simulink model "ifk_updated_armpi_fpv"  (R2023b)
settings: Solver=VariableStepAuto  StartTime=0.0001  StopTime=10.0  RelTol=1e-3
libraries: slpidlib x6
settings Model: Creator=15404  LastModifiedBy=PC
settings SolverCC: AlgebraicLoopSolver=TrustRegion
settings DebuggingCC: UnconnectedInputMsg=warning  UnconnectedOutputMsg=warning  UnconnectedLineMsg=warning
settings ModelReferenceCC: EnableRefExpFcnMdlSchedulingChecks=on
settings RTWCC: DLArmComputeVersion=19.05

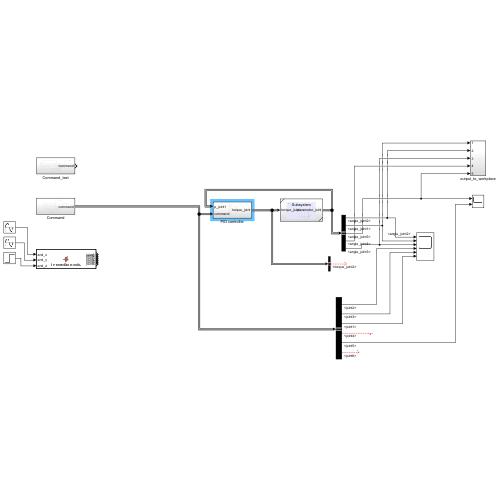
[thumbnail: Simulink's stored preview of the top-level diagram]
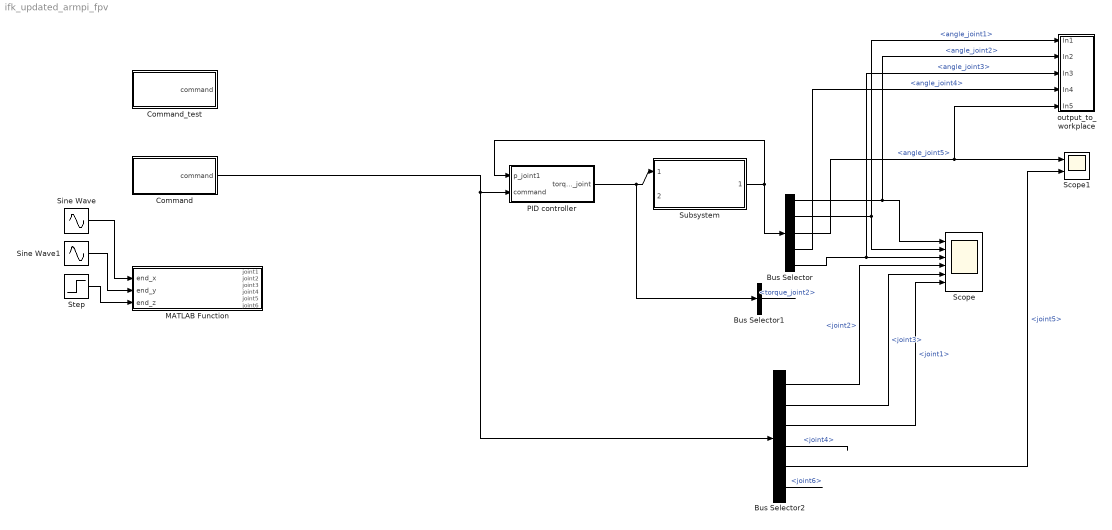
== system ifk_updated_armpi_fpv ==
  Bus Selector : BusSelector  OutputSignals=angle_joint2,angle_joint1,angle_joint5,angle_joint4,angle_joint3
  Bus Selector1 : BusSelector  OutputSignals=torque_joint2
  Bus Selector2 : BusSelector  OutputSignals=joint2,joint3,joint1,joint4,joint5,joint6
  Command : Subsystem
  Command_test : Subsystem
  MATLAB Function : MATLAB Function  TreatAsAtomicUnit=on
  PID controller : Subsystem
  Scope : Scope  NumInputPorts=6
  Scope1 : Scope  NumInputPorts=2
  Sine Wave : Sin  Amplitude=0.2  Phase=pi/2  SampleTime=0
  Sine Wave1 : Sin  Amplitude=0.2  SampleTime=0
  Step : Step  Time=0  After=0.1  SampleTime=0
  Subsystem : Subsystem  ReferencedSubsystem=Subsystem
  output_to_workplace : Subsystem
  wires:
  PID controller/1(torque_joint) -> Bus Selector1/1, Subsystem/1
  Subsystem/1 -> Bus Selector/1, PID controller/1(p_joint1)
  Bus Selector/1 -> output_to_workplace/2(In2), Scope/1  "<angle_joint2>"
  Bus Selector1/1 -> ?  "<torque_joint2>"
  Bus Selector/2 -> Scope/2, output_to_workplace/1(In1)  "<angle_joint1>"
  Bus Selector/3 -> output_to_workplace/5(In5), Scope1/1  "<angle_joint5>"
  Bus Selector/5 -> output_to_workplace/3(In3), Scope/3  "<angle_joint3>"
  Command/1(command) -> Bus Selector2/1, PID controller/2(command)
  Bus Selector2/1 -> Scope/4  "<joint2>"
  Bus Selector2/2 -> Scope/5  "<joint3>"
  Bus Selector2/3 -> Scope/6  "<joint1>"
  Bus Selector/4 -> output_to_workplace/4(In4)  "<angle_joint4>"
  Bus Selector2/4 -> ?  "<joint4>"
  Bus Selector2/5 -> Scope1/2  "<joint5>"
  Step/1 -> MATLAB Function/3(end_z)
  Sine Wave1/1 -> MATLAB Function/2(end_y)
  Sine Wave/1 -> MATLAB Function/1(end_x)
  Bus Selector2/6 -> ?  "<joint6>"

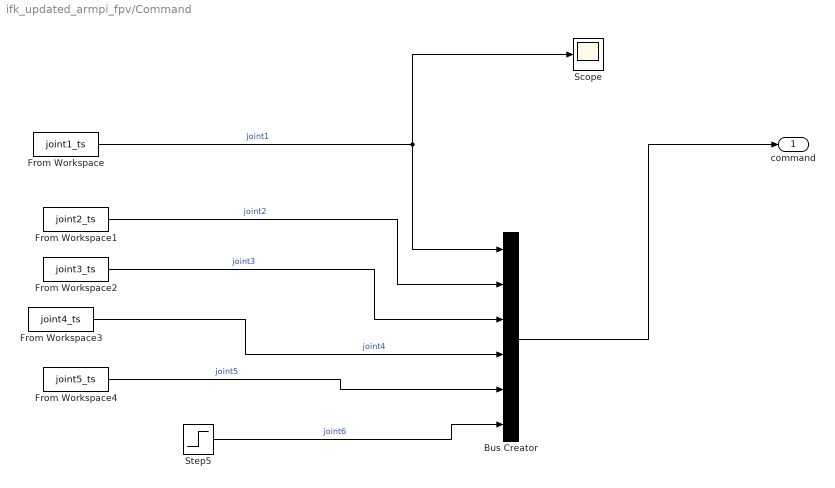
== system ifk_updated_armpi_fpv/Command ==
  Bus Creator : BusCreator  Inputs=6
  From Workspace : FromWorkspace  VariableName=joint1_ts
  From Workspace1 : FromWorkspace  VariableName=joint2_ts
  From Workspace2 : FromWorkspace  VariableName=joint3_ts
  From Workspace3 : FromWorkspace  VariableName=joint4_ts
  From Workspace4 : FromWorkspace  VariableName=joint5_ts
  Scope : Scope
  Step5 : Step  After=0  SampleTime=0
  command : Outport
  wires:
  Bus Creator/1 -> command/1
  From Workspace/1 -> Scope/1, Bus Creator/1  "joint1"
  From Workspace2/1 -> Bus Creator/3  "joint3"
  From Workspace3/1 -> Bus Creator/4  "joint4"
  From Workspace4/1 -> Bus Creator/5  "joint5"
  Step5/1 -> Bus Creator/6  "joint6"
  From Workspace1/1 -> Bus Creator/2  "joint2"

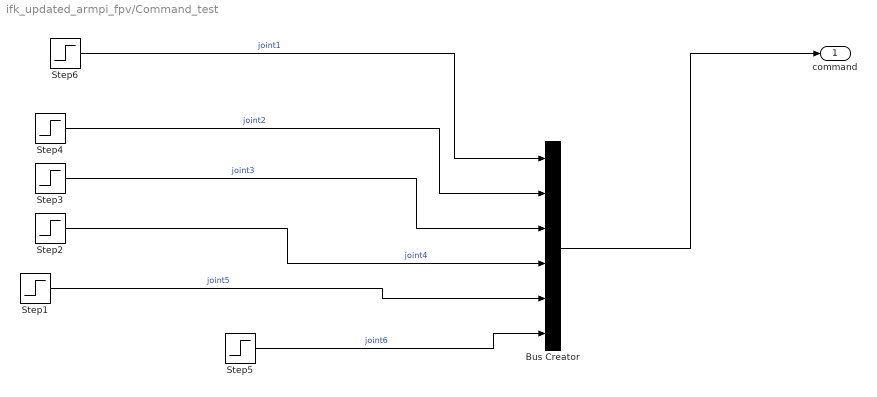
== system ifk_updated_armpi_fpv/Command_test ==
  Bus Creator : BusCreator  Inputs=6
  Step{1..6} (6 alike) : Step  After=0*pi/180  SampleTime=0
  command : Outport
  wires:
  Bus Creator/1 -> command/1
  Step6/1 -> Bus Creator/1  "joint1"
  Step3/1 -> Bus Creator/3  "joint3"
  Step2/1 -> Bus Creator/4  "joint4"
  Step1/1 -> Bus Creator/5  "joint5"
  Step5/1 -> Bus Creator/6  "joint6"
  Step4/1 -> Bus Creator/2  "joint2"

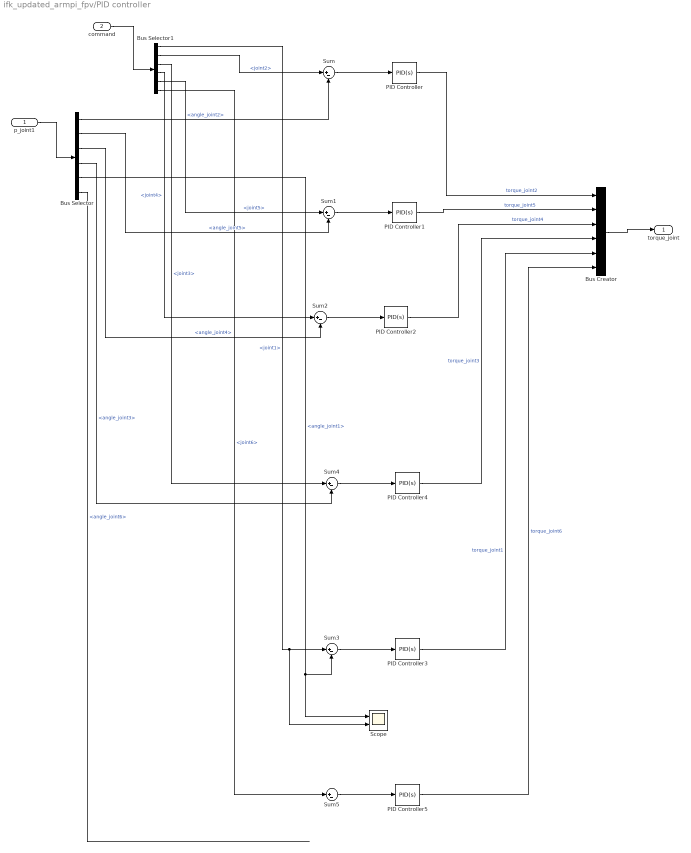
== system ifk_updated_armpi_fpv/PID controller ==
  p_joint1 : Inport
  command : Inport  Port=2
  Bus Creator : BusCreator  Inputs=6
  Bus Selector : BusSelector  OutputSignals=angle_joint2,angle_joint5,angle_joint4,angle_joint3,angle_joint1,angle_joint6
  Bus Selector1 : BusSelector  OutputSignals=joint1,joint2,joint3,joint4,joint5,joint6
  PID Controller : slpidlib/PID Controller  Controller=PID  Form=Parallel  TimeDomain=Continuous-time  UseExternalTs=off  SampleTime=-1  IntegratorMethod=Forward Euler  FilterMethod=Forward Euler  ControllerParametersSource=internal  P=5  I=500  UseKiTs=off  D=0.1  N=100  UseFilter=on  TunerSelectOption=Transfer Function Based (PID Tuner App)  InitialConditionSource=internal  InitialConditionForIntegrator=0  InitialConditionForFilter=0  DifferentiatorICPrevScaledInput=0  ExternalReset=none  TrackingMode=off  Kt=1  LimitOutput=off  SatLimitsSource=internal  UpperSaturationLimit=inf  LowerSaturationLimit=-inf  LinearizeAsGain=on  AntiWindupMode=none  Kb=1  LimitIntegrator=off  UpperIntegratorSaturationLimit=inf  LowerIntegratorSaturationLimit=-inf  POutMin=[]  POutMax=[]  IOutMin=[]  IOutMax=[]  DOutMin=[]  DOutMax=[]  NOutMin=[]  NOutMax=[]  SumOutMin=[]  SumOutMax=[]  SaturationOutMin=[]  SaturationOutMax=[]  PParamMin=[]  PParamMax=[]  IParamMin=[]  IParamMax=[]  DParamMin=[]  DParamMax=[]  NParamMin=[]  NParamMax=[]  KbParamMin=[]  KbParamMax=[]  KtParamMin=[]  KtParamMax=[]  KbOutMin=[]  KbOutMax=[]  KtOutMin=[]  KtOutMax=[]  IntegratorOutMin=[]  IntegratorOutMax=[]  FilterOutMin=[]  FilterOutMax=[]  SumI1OutMin=[]  SumI1OutMax=[]  SumI2OutMin=[]  SumI2OutMax=[]  SumI3OutMin=[]  SumI3OutMax=[]  SumI4OutMin=[]  SumI4OutMax=[]  SumDOutMin=[]  SumDOutMax=[]  DifferentiatorOutMin=[]  DifferentiatorOutMax=[]  FilterDiffOutCoefMin=[]  FilterDiffOutCoefMax=[]  ReciprocalOutMin=[]  ReciprocalOutMax=[]  SumDenOutMin=[]  SumDenOutMax=[]  SumNumOutMin=[]  SumNumOutMax=[]  DivideOutMin=[]  DivideOutMax=[]  UdiffTsProdOutMin=[]  UdiffTsProdOutMax=[]  NTsProdOutMin=[]  NTsProdOutMax=[]  UintegralTsProdOutMin=[]  UintegralTsProdOutMax=[]  UngainTsProdOutMin=[]  UngainTsProdOutMax=[]  ClampingZeroOutDataTypeStr=Inherit: Inherit via back propagation  ClampingZeroOutMin=[]  ClampingZeroOutMax=[]  FilterDenConstantOutDataTypeStr=Inherit: Inherit via back propagation  FilterDenConstantOutMin=[]  FilterDenConstantOutMax=[]  PCopyOutDataTypeStr=Inherit: Inherit via back propagation  PCopyOutMin=[]  PCopyOutMax=[]  NCopyOutDataTypeStr=Inherit: Inherit via back propagation  NCopyOutMin=[]  NCopyOutMax=[]  IntegratorContinuousStateAttributes=''  IntegratorStateMustResolveToSignalObject=off  IntegratorRTWStateStorageClass=Auto  FilterContinuousStateAttributes=''  FilterStateMustResolveToSignalObject=off  FilterRTWStateStorageClass=Auto  ParallelPVariant=InternalParameters  IdealPVariant=Disabled  IVariant=InternalParameters  DVariant=InternalParameters  IntegratorVariant=Continuous  SatVariant=Disabled  AWVariant=Passthrough  PCopyVariant=Disabled  TRVariant=Disabled  FdbkBlocksVariant=Forward  IdealPFdbkVariant=Disabled  SatFdbkVariant=Disabled  DerivativeFilterVariant=ContFilter  NVariant=InternalParameters  NCopyVariant=Disabled  FilterICVariant=InternalICsFilter  IntegratorICVariant=InternalICs  ExternalResetVariant=Disabled  TRSumVariant=Passthrough  SumFdbkVariant=Disabled  SumVariant=Sum_PID  TsampFilterVariant=InternalTs  TsampNgainVariant=Passthrough  TsampIntegralVariant=Disabled_SignalSpec  ExternalSaturationOutDataTypeStr=Inherit: Same as second input
  PID Controller{1..4} (4 alike) : slpidlib/PID Controller  Controller=PID  Form=Parallel  TimeDomain=Continuous-time  UseExternalTs=off  SampleTime=-1  IntegratorMethod=Forward Euler  FilterMethod=Forward Euler  ControllerParametersSource=internal  P=1  I=50  UseKiTs=off  D=0.1  N=100  UseFilter=on  TunerSelectOption=Transfer Function Based (PID Tuner App)  InitialConditionSource=internal  InitialConditionForIntegrator=0  InitialConditionForFilter=0  DifferentiatorICPrevScaledInput=0  ExternalReset=none  TrackingMode=off  Kt=1  LimitOutput=off  SatLimitsSource=internal  UpperSaturationLimit=inf  LowerSaturationLimit=-inf  LinearizeAsGain=on  AntiWindupMode=none  Kb=1  LimitIntegrator=off  UpperIntegratorSaturationLimit=inf  LowerIntegratorSaturationLimit=-inf  POutMin=[]  POutMax=[]  IOutMin=[]  IOutMax=[]  DOutMin=[]  DOutMax=[]  NOutMin=[]  NOutMax=[]  SumOutMin=[]  SumOutMax=[]  SaturationOutMin=[]  SaturationOutMax=[]  PParamMin=[]  PParamMax=[]  IParamMin=[]  IParamMax=[]  DParamMin=[]  DParamMax=[]  NParamMin=[]  NParamMax=[]  KbParamMin=[]  KbParamMax=[]  KtParamMin=[]  KtParamMax=[]  KbOutMin=[]  KbOutMax=[]  KtOutMin=[]  KtOutMax=[]  IntegratorOutMin=[]  IntegratorOutMax=[]  FilterOutMin=[]  FilterOutMax=[]  SumI1OutMin=[]  SumI1OutMax=[]  SumI2OutMin=[]  SumI2OutMax=[]  SumI3OutMin=[]  SumI3OutMax=[]  SumI4OutMin=[]  SumI4OutMax=[]  SumDOutMin=[]  SumDOutMax=[]  DifferentiatorOutMin=[]  DifferentiatorOutMax=[]  FilterDiffOutCoefMin=[]  FilterDiffOutCoefMax=[]  ReciprocalOutMin=[]  ReciprocalOutMax=[]  SumDenOutMin=[]  SumDenOutMax=[]  SumNumOutMin=[]  SumNumOutMax=[]  DivideOutMin=[]  DivideOutMax=[]  UdiffTsProdOutMin=[]  UdiffTsProdOutMax=[]  NTsProdOutMin=[]  NTsProdOutMax=[]  UintegralTsProdOutMin=[]  UintegralTsProdOutMax=[]  UngainTsProdOutMin=[]  UngainTsProdOutMax=[]  ClampingZeroOutDataTypeStr=Inherit: Inherit via back propagation  ClampingZeroOutMin=[]  ClampingZeroOutMax=[]  FilterDenConstantOutDataTypeStr=Inherit: Inherit via back propagation  FilterDenConstantOutMin=[]  FilterDenConstantOutMax=[]  PCopyOutDataTypeStr=Inherit: Inherit via back propagation  PCopyOutMin=[]  PCopyOutMax=[]  NCopyOutDataTypeStr=Inherit: Inherit via back propagation  NCopyOutMin=[]  NCopyOutMax=[]  IntegratorContinuousStateAttributes=''  IntegratorStateMustResolveToSignalObject=off  IntegratorRTWStateStorageClass=Auto  FilterContinuousStateAttributes=''  FilterStateMustResolveToSignalObject=off  FilterRTWStateStorageClass=Auto  ParallelPVariant=InternalParameters  IdealPVariant=Disabled  IVariant=InternalParameters  DVariant=InternalParameters  IntegratorVariant=Continuous  SatVariant=Disabled  AWVariant=Passthrough  PCopyVariant=Disabled  TRVariant=Disabled  FdbkBlocksVariant=Forward  IdealPFdbkVariant=Disabled  SatFdbkVariant=Disabled  DerivativeFilterVariant=ContFilter  NVariant=InternalParameters  NCopyVariant=Disabled  FilterICVariant=InternalICsFilter  IntegratorICVariant=InternalICs  ExternalResetVariant=Disabled  TRSumVariant=Passthrough  SumFdbkVariant=Disabled  SumVariant=Sum_PID  TsampFilterVariant=InternalTs  TsampNgainVariant=Passthrough  TsampIntegralVariant=Disabled_SignalSpec  ExternalSaturationOutDataTypeStr=Inherit: Same as second input
  PID Controller5 : slpidlib/PID Controller  Controller=PID  Form=Parallel  TimeDomain=Continuous-time  UseExternalTs=off  SampleTime=-1  IntegratorMethod=Forward Euler  FilterMethod=Forward Euler  ControllerParametersSource=internal  P=1  I=5  UseKiTs=off  D=1  N=100  UseFilter=on  TunerSelectOption=Transfer Function Based (PID Tuner App)  InitialConditionSource=internal  InitialConditionForIntegrator=0  InitialConditionForFilter=0  DifferentiatorICPrevScaledInput=0  ExternalReset=none  TrackingMode=off  Kt=1  LimitOutput=off  SatLimitsSource=internal  UpperSaturationLimit=inf  LowerSaturationLimit=-inf  LinearizeAsGain=on  AntiWindupMode=none  Kb=1  LimitIntegrator=off  UpperIntegratorSaturationLimit=inf  LowerIntegratorSaturationLimit=-inf  POutMin=[]  POutMax=[]  IOutMin=[]  IOutMax=[]  DOutMin=[]  DOutMax=[]  NOutMin=[]  NOutMax=[]  SumOutMin=[]  SumOutMax=[]  SaturationOutMin=[]  SaturationOutMax=[]  PParamMin=[]  PParamMax=[]  IParamMin=[]  IParamMax=[]  DParamMin=[]  DParamMax=[]  NParamMin=[]  NParamMax=[]  KbParamMin=[]  KbParamMax=[]  KtParamMin=[]  KtParamMax=[]  KbOutMin=[]  KbOutMax=[]  KtOutMin=[]  KtOutMax=[]  IntegratorOutMin=[]  IntegratorOutMax=[]  FilterOutMin=[]  FilterOutMax=[]  SumI1OutMin=[]  SumI1OutMax=[]  SumI2OutMin=[]  SumI2OutMax=[]  SumI3OutMin=[]  SumI3OutMax=[]  SumI4OutMin=[]  SumI4OutMax=[]  SumDOutMin=[]  SumDOutMax=[]  DifferentiatorOutMin=[]  DifferentiatorOutMax=[]  FilterDiffOutCoefMin=[]  FilterDiffOutCoefMax=[]  ReciprocalOutMin=[]  ReciprocalOutMax=[]  SumDenOutMin=[]  SumDenOutMax=[]  SumNumOutMin=[]  SumNumOutMax=[]  DivideOutMin=[]  DivideOutMax=[]  UdiffTsProdOutMin=[]  UdiffTsProdOutMax=[]  NTsProdOutMin=[]  NTsProdOutMax=[]  UintegralTsProdOutMin=[]  UintegralTsProdOutMax=[]  UngainTsProdOutMin=[]  UngainTsProdOutMax=[]  ClampingZeroOutDataTypeStr=Inherit: Inherit via back propagation  ClampingZeroOutMin=[]  ClampingZeroOutMax=[]  FilterDenConstantOutDataTypeStr=Inherit: Inherit via back propagation  FilterDenConstantOutMin=[]  FilterDenConstantOutMax=[]  PCopyOutDataTypeStr=Inherit: Inherit via back propagation  PCopyOutMin=[]  PCopyOutMax=[]  NCopyOutDataTypeStr=Inherit: Inherit via back propagation  NCopyOutMin=[]  NCopyOutMax=[]  IntegratorContinuousStateAttributes=''  IntegratorStateMustResolveToSignalObject=off  IntegratorRTWStateStorageClass=Auto  FilterContinuousStateAttributes=''  FilterStateMustResolveToSignalObject=off  FilterRTWStateStorageClass=Auto  ParallelPVariant=InternalParameters  IdealPVariant=Disabled  IVariant=InternalParameters  DVariant=InternalParameters  IntegratorVariant=Continuous  SatVariant=Disabled  AWVariant=Passthrough  PCopyVariant=Disabled  TRVariant=Disabled  FdbkBlocksVariant=Forward  IdealPFdbkVariant=Disabled  SatFdbkVariant=Disabled  DerivativeFilterVariant=ContFilter  NVariant=InternalParameters  NCopyVariant=Disabled  FilterICVariant=InternalICsFilter  IntegratorICVariant=InternalICs  ExternalResetVariant=Disabled  TRSumVariant=Passthrough  SumFdbkVariant=Disabled  SumVariant=Sum_PID  TsampFilterVariant=InternalTs  TsampNgainVariant=Passthrough  TsampIntegralVariant=Disabled_SignalSpec  ExternalSaturationOutDataTypeStr=Inherit: Same as second input
  Scope : Scope  NumInputPorts=2
  Sum{,1..5} (6 alike) : Sum  Inputs=|+-
  torque_joint : Outport
  wires:
  p_joint1/1 -> Bus Selector/1
  Bus Selector/1 -> Sum/2  "<angle_joint2>"
  Sum/1 -> PID Controller/1
  PID Controller/1 -> Bus Creator/1  "torque_joint2"
  PID Controller1/1 -> Bus Creator/2  "torque_joint5"
  Sum1/1 -> PID Controller1/1
  Bus Selector/2 -> Sum1/2  "<angle_joint5>"
  Bus Selector/4 -> Sum4/2  "<angle_joint3>"
  Bus Selector/5 -> Scope/1, Sum3/2  "<angle_joint1>"
  Bus Selector/3 -> Sum2/2  "<angle_joint4>"
  PID Controller2/1 -> Bus Creator/3  "torque_joint4"
  Sum2/1 -> PID Controller2/1
  Sum3/1 -> PID Controller3/1
  PID Controller3/1 -> Bus Creator/5  "torque_joint1"
  command/1 -> Bus Selector1/1
  PID Controller4/1 -> Bus Creator/4  "torque_joint3"
  Sum4/1 -> PID Controller4/1
  Bus Creator/1 -> torque_joint/1
  Bus Selector1/1 -> Scope/2, Sum3/1  "<joint1>"
  Bus Selector1/2 -> Sum/1  "<joint2>"
  Bus Selector1/5 -> Sum1/1  "<joint5>"
  Bus Selector1/3 -> Sum4/1  "<joint3>"
  Bus Selector1/4 -> Sum2/1  "<joint4>"
  Sum5/1 -> PID Controller5/1
  Bus Selector1/6 -> Sum5/1  "<joint6>"
  Bus Selector/6 -> ?  "<angle_joint6>"
  PID Controller5/1 -> Bus Creator/6  "torque_joint6"

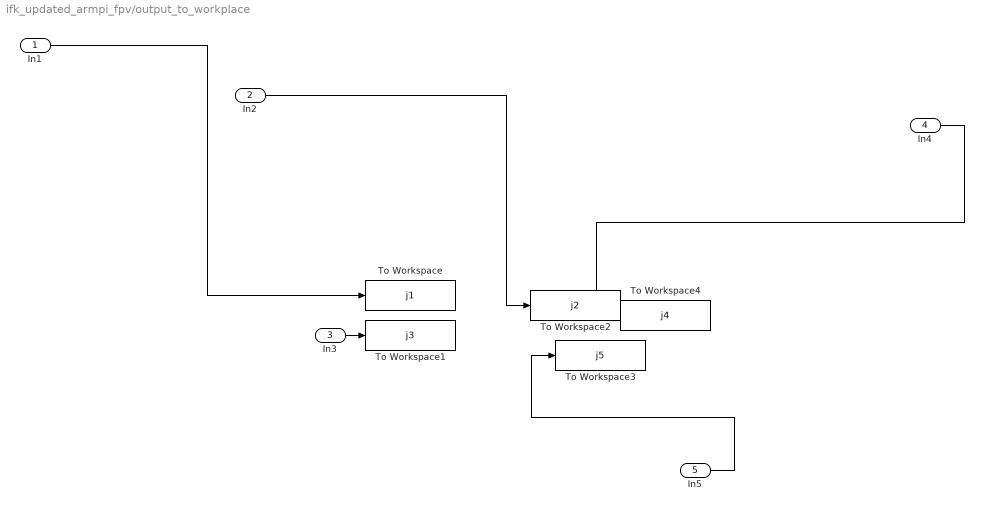
== system ifk_updated_armpi_fpv/output_to_workplace ==
  In1 : Inport
  In2 : Inport  Port=2
  In3 : Inport  Port=3
  In4 : Inport  Port=4
  In5 : Inport  Port=5
  To Workspace : ToWorkspace  VariableName=j1  SaveFormat=Timeseries  SampleTime=-1
  To Workspace1 : ToWorkspace  VariableName=j3  SaveFormat=Timeseries  SampleTime=-1
  To Workspace2 : ToWorkspace  VariableName=j2  SaveFormat=Timeseries  SampleTime=-1
  To Workspace3 : ToWorkspace  VariableName=j5  SaveFormat=Timeseries  SampleTime=-1
  To Workspace4 : ToWorkspace  VariableName=j4  SaveFormat=Timeseries  SampleTime=-1
  wires:
  In2/1 -> To Workspace2/1
  In4/1 -> To Workspace4/1
  In5/1 -> To Workspace3/1
  In1/1 -> To Workspace/1
  In3/1 -> To Workspace1/1

== matlab function ifk_updated_armpi_fpv/MATLAB Function ==
  data: end_x input; joint1 output; end_y input; end_z input; joint2 output; joint3 output; joint4 output; joint5 output; joint6 output
function [joint1,joint2,joint3,joint4,joint5,joint6] = InverseKenimatic(end_x,end_y,end_z)

coder.extrinsic('load_system')


% 
% targets = [end_x,end_y,end_z];
% [outputVec,statusFlag] = solve(ik,targets);
% joint1 = outputVec(1);
% joint2 = outputVec(2);
% joint3 = outputVec(3);
% joint4 = outputVec(4);
% joint5 = outputVec(5);
% joint6 = 0;

joint1 = 0;
joint2 = 0;
joint3 = 0;
joint4 = 0;
joint5 = 0;
joint6 = 0;
